simulink model "Quadcopter_ControllerWithNavigation"  (R2024b)
settings: Solver=FixedStepAuto  StartTime=0.0  StopTime=inf  RelTol=1e-3  EnableMultiTasking=on
undefined symbols (not defined in the file): SampleTime
libraries: px4uORBlib x10, slpidlib x10, simulink x4, uavalgslib x3, px4Utilslib x2, px4Peripheralslib x1, simulink_extras x1, sharedutil x1, sharedtransform x1
(part 3 of 3)

== system Quadcopter_ControllerWithNavigation/Navigation/Quadcopter Navigation Algorithm/Read waypoint from QGroundControl Mission/Guidance Subsystem/Land/Maintain Current Yaw during Land ==
  yaw_In : Inport
  Constant : Constant  Value=0
  Delay : Delay  DelayLength=1  InitialCondition=1
  Enabled Subsystem2 : Subsystem  TreatAsAtomicUnit=on
  yaw_Out : Outport
  wires:
  Delay/1 -> Enabled Subsystem2/Enable
  Constant/1 -> Delay/1
  yaw_In/1 -> Enabled Subsystem2/1(yaw_In)
  Enabled Subsystem2/1(yaw_Out) -> yaw_Out/1

== system Quadcopter_ControllerWithNavigation/Navigation/Quadcopter Navigation Algorithm/Read waypoint from QGroundControl Mission/Guidance Subsystem/Take-off/Ensure smooth ascend during Takeoff ==
  In1 : Inport
  Delay : Delay  DelayLength=1
  Gain : Gain  Gain=-1
  Gain1 : Gain  Gain=-1
  Rate : Constant  Value=0.01
  Relational Operator : RelationalOperator  Operator=<=  OutDataTypeStr=boolean  RndMeth=Simplest  InputSameDT=off
  Sum : Sum  Inputs=|++
  Switch : Switch  Criteria=u2 > Threshold  SaturateOnIntegerOverflow=off  InputSameDT=off
  Out1 : Outport
  wires:
  Rate/1 -> Sum/1
  Gain/1 -> Out1/1
  Relational Operator/1 -> Switch/2
  Switch/1 -> Gain/1
  In1/1 -> Gain1/1
  Sum/1 -> Relational Operator/2, Switch/3, Delay/1
  Gain1/1 -> Switch/1, Relational Operator/1
  Delay/1 -> Sum/2

== system Quadcopter_ControllerWithNavigation/Navigation/Quadcopter Navigation Algorithm/Read waypoint from QGroundControl Mission/Guidance Subsystem/Take-off/Maintain Current Yaw during TakeOff ==
  yaw_In : Inport
  Constant : Constant  Value=0
  Delay : Delay  DelayLength=1  InitialCondition=1
  Enabled Subsystem2 : Subsystem  TreatAsAtomicUnit=on
  yaw_Out : Outport
  wires:
  yaw_In/1 -> Enabled Subsystem2/1(yaw_In)
  Enabled Subsystem2/1(yaw_Out) -> yaw_Out/1
  Delay/1 -> Enabled Subsystem2/Enable
  Constant/1 -> Delay/1

== system Quadcopter_ControllerWithNavigation/Navigation/Quadcopter Navigation Algorithm/Read waypoint from QGroundControl Mission/Guidance Subsystem/Waypoint/Output signal conditioning ==
  Current Position : Inport
  LookAhead Point : Inport  Port=2
  Desired Yaw : Inport  Port=3
  Waypoint Type : Inport  Port=4
  Compare To Constant : simulink/Logic and Bit Operations/Compare To Constant  relop===  const=5  OutDataTypeStr=boolean
  Constant : Constant  Value=0  SampleTime=-1
  IsNaN : RelationalOperator  Operator=isNaN  OutDataTypeStr=boolean  RndMeth=Simplest  InputSameDT=off
  IsNaN1 : RelationalOperator  Operator=isNaN  OutDataTypeStr=boolean  RndMeth=Simplest  InputSameDT=off
  Matrix Concatenate1 : Concatenate  Mode=Multidimensional array  ConcatenateDimension=2
  OR : Logic  Operator=OR  IconShape=distinctive  AllPortsSameDT=off  OutDataTypeStr=boolean
  OR1 : Logic  Operator=OR  Inputs=1  IconShape=distinctive  AllPortsSameDT=off  OutDataTypeStr=boolean
  Reshape2 : Reshape  OutputDimensionality=Row vector (2-D)
  Reshape3 : Reshape  OutputDimensionality=Row vector (2-D)
  Switch : Switch  Criteria=u2 ~= 0  SaturateOnIntegerOverflow=off  InputSameDT=off
  Switch1 : Switch  Criteria=u2 > Threshold  SaturateOnIntegerOverflow=off  InputSameDT=off
  Transpose1 : Math  Operator=transpose
  xyzYaw : Outport
  wires:
  IsNaN1/1 -> OR1/1
  Reshape2/1 -> Matrix Concatenate1/2
  Matrix Concatenate1/1 -> Switch1/3
  OR/1 -> Switch1/2
  LookAhead Point/1 -> IsNaN1/1, Transpose1/1
  Compare To Constant/1 -> OR/2
  Transpose1/1 -> Matrix Concatenate1/1
  IsNaN/1 -> Switch/2
  Reshape3/1 -> Switch1/1
  Waypoint Type/1 -> Compare To Constant/1
  Switch1/1 -> xyzYaw/1
  Current Position/1 -> Reshape3/1
  OR1/1 -> OR/1
  Constant/1 -> Switch/1
  Switch/1 -> Reshape2/1
  Desired Yaw/1 -> Switch/3, IsNaN/1

== system Quadcopter_ControllerWithNavigation/Navigation/Quadcopter Navigation Algorithm/Path Correction from Onboard Computer/Guidance Subsystem/IDLE/Maintain Current Yaw during IDLE/Enabled Subsystem2 ==
  yaw_In : Inport
  Enable : EnablePort
  yaw_Out : Outport
  wires:
  yaw_In/1 -> yaw_Out/1

== system Quadcopter_ControllerWithNavigation/Navigation/Quadcopter Navigation Algorithm/Path Correction from Onboard Computer/Guidance Subsystem/Land/Ensure Smooth descend during Land/Enabled Subsystem ==
  In : Inport
  Enable : EnablePort
  Out : Outport
  wires:
  In/1 -> Out/1

== system Quadcopter_ControllerWithNavigation/Navigation/Quadcopter Navigation Algorithm/Path Correction from Onboard Computer/Guidance Subsystem/Land/Maintain Current Yaw during Land/Enabled Subsystem2 ==
  yaw_In : Inport
  Enable : EnablePort
  yaw_Out : Outport
  wires:
  yaw_In/1 -> yaw_Out/1

== system Quadcopter_ControllerWithNavigation/Navigation/Quadcopter Navigation Algorithm/Path Correction from Onboard Computer/Guidance Subsystem/Take-off/Maintain Current Yaw during TakeOff/Enabled Subsystem2 ==
  yaw_In : Inport
  Enable : EnablePort
  yaw_Out : Outport
  wires:
  yaw_In/1 -> yaw_Out/1

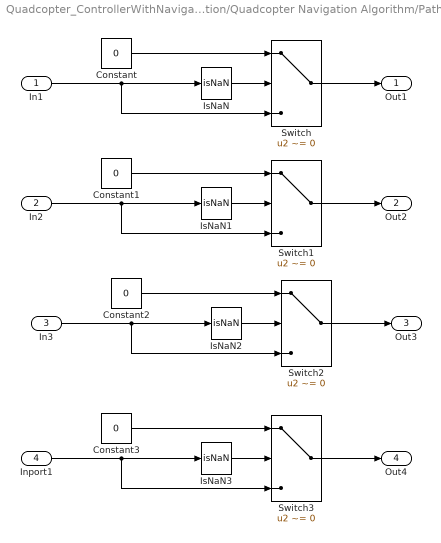
== system Quadcopter_ControllerWithNavigation/Navigation/Quadcopter Navigation Algorithm/Path Correction from Onboard Computer/Guidance Subsystem/Waypoint/Waypoints/NAN check ==
  In1 : Inport
  In2 : Inport  Port=2
  In3 : Inport  Port=3
  Inport1 : Inport  Port=4
  Constant{,1..3} (4 alike) : Constant  Value=0  SampleTime=-1
  IsNaN{,1..3} (4 alike) : RelationalOperator  Operator=isNaN  OutDataTypeStr=boolean  RndMeth=Simplest  InputSameDT=off
  Switch{,1..3} (4 alike) : Switch  Criteria=u2 ~= 0  SaturateOnIntegerOverflow=off  InputSameDT=off
  Out1 : Outport
  Out2 : Outport  Port=2
  Out3 : Outport  Port=3
  Out4 : Outport  Port=4
  wires:
  Switch/1 -> Out1/1
  In1/1 -> Switch/3, IsNaN/1
  Constant/1 -> Switch/1
  IsNaN/1 -> Switch/2
  Switch1/1 -> Out2/1
  IsNaN1/1 -> Switch1/2
  In2/1 -> Switch1/3, IsNaN1/1
  Constant1/1 -> Switch1/1
  Switch2/1 -> Out3/1
  IsNaN2/1 -> Switch2/2
  In3/1 -> Switch2/3, IsNaN2/1
  Constant2/1 -> Switch2/1
  Inport1/1 -> Switch3/3, IsNaN3/1
  Switch3/1 -> Out4/1
  Constant3/1 -> Switch3/1
  IsNaN3/1 -> Switch3/2

== system Quadcopter_ControllerWithNavigation/Navigation/Quadcopter Navigation Algorithm/Read waypoint from QGroundControl Mission/Guidance Subsystem/IDLE/Maintain Current Yaw during IDLE/Enabled Subsystem2 ==
  yaw_In : Inport
  Enable : EnablePort
  yaw_Out : Outport
  wires:
  yaw_In/1 -> yaw_Out/1

== system Quadcopter_ControllerWithNavigation/Navigation/Quadcopter Navigation Algorithm/Read waypoint from QGroundControl Mission/Guidance Subsystem/Land/Ensure Smooth descend during Land/Enabled Subsystem ==
  In : Inport
  Enable : EnablePort
  Out : Outport
  wires:
  In/1 -> Out/1

== system Quadcopter_ControllerWithNavigation/Navigation/Quadcopter Navigation Algorithm/Read waypoint from QGroundControl Mission/Guidance Subsystem/Land/Maintain Current Yaw during Land/Enabled Subsystem2 ==
  yaw_In : Inport
  Enable : EnablePort
  yaw_Out : Outport
  wires:
  yaw_In/1 -> yaw_Out/1

== system Quadcopter_ControllerWithNavigation/Navigation/Quadcopter Navigation Algorithm/Read waypoint from QGroundControl Mission/Guidance Subsystem/Take-off/Maintain Current Yaw during TakeOff/Enabled Subsystem2 ==
  yaw_In : Inport
  Enable : EnablePort
  yaw_Out : Outport
  wires:
  yaw_In/1 -> yaw_Out/1

== matlab function Quadcopter_ControllerWithNavigation/MATLAB Function1 ==
  data: x input; label output
function label = classifyManually(x)
% x: vettore [10x1] di tipo single

if x(3) < 1503.13
    if x(1) < 0.247179
        label = 0;
    else
        label = 1105;
    end
else
    if x(2) < 1568.93
        if x(2) < 1536.56
            label = 1105;
        else
            label = 1110;
        end
    else
        label = 1115;
    end
end

label = double(label);  % per code generation embedded

== matlab function Quadcopter_ControllerWithNavigation/MATLAB Function ==
  data: featureVector output; fy input; fa input
function featureVector = featureGenerate_top10(fy, fa)
% Calcola le 10 feature derivate dal Diagnostic Feature Designer
% fx = acc_x_reale
% fy = acc_y_reale
% fa = actuator_1
% fr = res_y
% Tutti sono buffer (Nx1 vettori)
% Output: featureVector (1x10)

% 'omnitan' e 'rms' NON sono supportati nella conversione in C.

% Feature 1: acc_x_reale_sigstats/Std
%f1 = std(fx);

% Feature 2-5: acc_y_reale_sigstats/Mean, PeakValue, RMS, Std
%f2 = mean(fy);
f3 = max(abs(fy));
%f4 = rms(fy, 'omitnan');
%f4 = sqrt(mean(fy.^2));  % equivalente a rms
%f5 = std(fy);

% Feature 6-8: actuator_1_sigstats/Mean, PeakValue, RMS
f6 = mean(fa);
% f7 = max(abs(fa));
%f8 = rms(fa, 'omitnan');
f8 = sqrt(mean(fa.^2));

% Feature 9-10: res_y_sigstats/PeakValue, Std
%f9 = max(abs(fr));
%f10 = std(fr);

% Output feature vector
%featureVector = single([f1 f2 f3 f4 f5 f6 f7 f8 f9 f10]');
featureVector = single([f3 f6 f8]');

== matlab function Quadcopter_ControllerWithNavigation/MATLAB Function2 ==
  data: fy input; label output; fa input
function label = predictMinimalBuffered(fy, fa)
% FY = acc_y_reale (singolo campione), FA = actuator_1 (singolo campione)
% Output: label (double) basato su classificazione su buffer

% Buffer persistente
persistent fyBuffer faBuffer

% Inizializzazione buffer a 128 elementi
if isempty(fyBuffer)
    fyBuffer = zeros(1, 500);
    faBuffer = zeros(1, 500);
end

% Sostituzione NaN con 0
if isnan(fy)
    fy = 0;
end
if isnan(fa)
    fa = 0;
end

% Aggiornamento buffer (FIFO)
fyBuffer = [fyBuffer(2:end), fy];
faBuffer = [faBuffer(2:end), fa];

% Calcolo feature direttamente su buffer aggiornato
if sqrt(mean(faBuffer.^2)) < 1503.13
    if mean(fyBuffer) < 0.247179
        label = 0;
    else
        label = 1105;
    end
else
    if mean(faBuffer) < 1568.93
        if mean(faBuffer) < 1536.56
            label = 1105;
        else
            label = 1110;
        end
    else
        label = 1115;
    end
end

label = double(label);  % per compatibilità con code generation
end

== matlab function Quadcopter_ControllerWithNavigation/MATLAB Function3 ==
  data: acc_y input; label output; act1 input; f1 output; f2 output; f3 output
function [label, f1, f2, f3] = classificatore(acc_y, act1) %#codegen
% acc_y, act1: vettori (1x128 o 128x1) contenenti i campioni del segnale
% Output: label (uint16) del classificatore; f1, f2, f3 feature calcolate

% Prealloca la variabile label
uint16 label;

% Imposta la dimensione del frame
frameSize = 128;
n = length(acc_y);

% Definisce gli indici per il frame corrente
startIdx = n - frameSize + 1;
endIdx = n;

% Estrae i segmenti di segnale per il frame corrente
frame_acc_y = acc_y(startIdx:endIdx);
frame_act1 = act1(startIdx:endIdx);

% Denormalizza il segnale PWM
frame_act1_denorm = frame_act1 * 1000 + 1000;

% Calcolo delle feature per acc_y
f1 = mean(frame_acc_y);                      % Media di acc_y

% Calcolo delle feature per act1
f2 = mean(frame_act1_denorm);                % Media di act1
f3 = sqrt(mean(frame_act1_denorm.^2));       % Valore RMS di act1

% Controllo: se il drone non sta effettivamente volando non esegue il classificatore
    if f2 <=1350
        label = -1;
        return
    end

% Classificazione basata sull'albero decisionale
    if f3 < 1503.13
        if f1 < 0.247179
            label = 0;
        else
            label = 1;
        end
    else
        if f2 < 1568.93
            if f2 < 1536.56
                label = 1;
            else
                label = 2;
            end
        else
            label = 3;
        end
    end
end

== matlab function Quadcopter_ControllerWithNavigation/MATLAB Function4 ==
  data: acc_y input; label output; act1 input
function label = featureGenerate_accY_act1(acc_y, act1) %#codegen

% VECCHIA FUNZIONE DEL 03/04/2025

% Imposta la dimensione del frame
frameSize = 128;
n = length(acc_y);

% Prealloca la variabile label
uint16 label;

% Definisci gli indici per il frame corrente
startIdx = n - frameSize + 1;
endIdx = n;

% Estrai i segmenti di segnale per il frame corrente
fy = acc_y(startIdx:endIdx);
fa = act1(startIdx:endIdx);

% Calcolo delle feature per acc_y
f1 = mean(fy);           % Media di acc_y

% Calcolo delle feature per act1
f5 = mean(fa);           % Media di act1
f7 = sqrt(mean(fa.^2));  % Valore RMS di act1

% Costruisci il classificatore
if f7 < 1503.13
    if f1 < 0.247179
        label = 0;
    else
        label = 1105;
    end
else
    if f5 < 1568.93
        if f5 < 1536.56
            label = 1105;
        else
            label = 1110;
        end
    else
        label = 1115;
    end
end
end

== matlab function Quadcopter_ControllerWithNavigation/MATLAB Function5 ==
  data: acc_x_reale input; acc_y_reale input; label output; act1 input; res_y input; f1 output; f2 output; f3 output; f4 output; f5 output; f6 output; f7 output
function [label, f1, f2, f3, f4, f5, f6, f7]  = classificatore(acc_x_reale, acc_y_reale, act1, res_y) %#codegen
    % acc_y_reale, act1, acc_x_reale, res_y: vettori (1x128 o 128x1) contenenti i campioni del segnale
    % Output: label (uint16) del classificatore; f1-f7 feature calcolate
    
    % Preallocazione
    uint16 label;
    
    % Dimensione del frame
    frameSize = 128;
    n = length(acc_y_reale);
    startIdx = n - frameSize + 1;
    endIdx = n;
    
    % Estrai i frame correnti
    frame_acc_y = acc_y_reale(startIdx:endIdx);
    frame_act1 = act1(startIdx:endIdx);
    frame_acc_x = acc_x_reale(startIdx:endIdx);
    frame_res_y = res_y(startIdx:endIdx);
    
    % Denormalizza act1
    frame_act1_denorm = frame_act1 * 1000 + 1000;
    
    % Calcolo feature
    f1 = mean(frame_acc_y);                          % acc_y Mean
    f2 = mean(frame_act1_denorm);                    % act1 Mean
    f3 = sqrt(mean(frame_act1_denorm.^2));           % act1 RMS
    f4 = max(frame_act1_denorm);                     % act1 PeakValue
    f5 = std(frame_acc_x);                           % acc_x Std
    f6 = max(frame_acc_y);                           % acc_y PeakValue
    f7 = max(frame_res_y);                           % res_y PeakValue
    
    % Controllo: se il drone non vola, skip
    if f2 <= 1350
        label = -1;  % codice speciale per 'non classificato'
        return
    end
    
    % Classificazione basata sul Medium Tree
    if f3 < 1503.13
        if f1 < 0.247179
            if f5 < 0.0155678
                if f1 < -0.0891853
                    label = 1;
                else
                    label = 0;
                end
            else
                if f1 < 0.050047
                    if f2 < 1487.41
                        label = 0;
                    else
                        label = 1;
                    end
                else
                    label = 0;
                end
            end
        else
            if f1 < 0.258214
                label = 2;
            else
                label = 1;
            end
        end
    else
        if f2 < 1568.93
            if f2 < 1536.56
                if f5 < 0.0175373
                    if f2 < 1524.54
                        label = 1;
                    else
                        label = 0;
                    end
                else
                    if f1 < 0.254381
                        label = 0;
                    else
                        label = 1;
                    end
                end
            else
                if f1 < 0.254912
                    label = 2;
                else
                    if f7 < 0.141758
                        label = 1;
                    else
                        label = 3;
                    end
                end
            end
        else
            if f4 < 1652.77
                if f5 < 0.0164272
                    label = 3;
                else
                    if f1 < -0.170482
                        label = 2;
                    else
                        label = 3;
                    end
                end
            else
                if f6 < 0.282649
                    if f1 < 0.0264928
                        label = 3;
                    else
                        label = 2;
                    end
                else
                    label = 3;
                end
            end
        end
    end
end
